simulink model "Fuel_Cell_System"  (R2024a)
settings: Solver=VariableStepAuto  StartTime=0.0  StopTime=10.0  RelTol=1e-3
undefined symbols (not defined in the file): A, Rload
libraries: fl_lib x9, ee_lib x2, nesl_utility x2
settings Model: Creator=Miko  LastModifiedBy=Miko

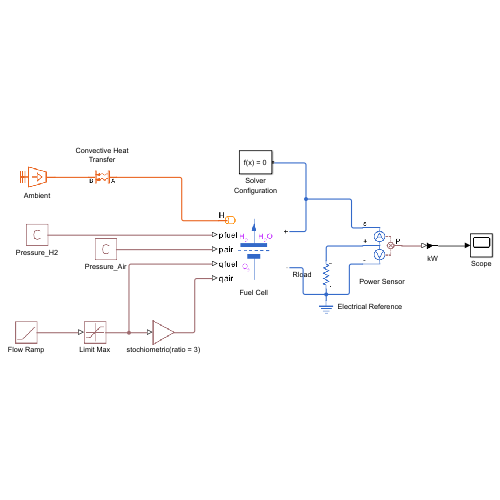
[thumbnail: Simulink's stored preview of the top-level diagram]
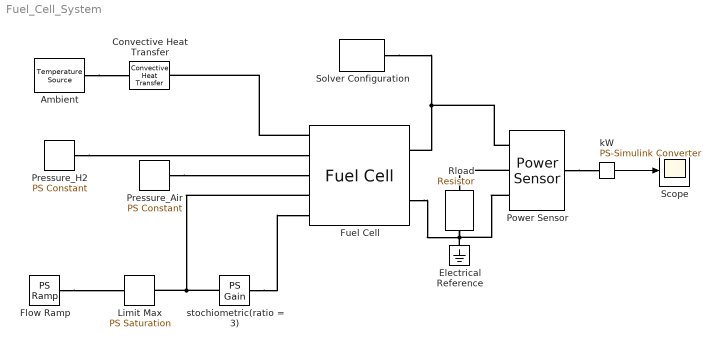
== system Fuel_Cell_System ==
  Ambient : fl_lib/Thermal/Thermal Sources/Temperature Source  temperature=293.15 K
  Convective Heat Transfer : fl_lib/Thermal/Thermal Elements/Convective Heat Transfer  thermal_type=foundation.enum.constant_variable.constant  area=120 cm^2  heat_tr_coeff=20 W/(K*m^2)  min_heat_tr_coeff=1e-3 W/(K*m^2)  T_specify=off  T_priority=None  T=0 K  T_nominal_specify=off  T_nominal_value=1  T_nominal_unit=K  Q_specify=off  Q_priority=None  Q=0 W  Q_nominal_specify=off  Q_nominal_value=1  Q_nominal_unit=W
  Electrical Reference : fl_lib/Electrical/Electrical Elements/Electrical Reference
  Flow Ramp : fl_lib/Physical Signals/Sources/PS Ramp  slope=100/60 lpm/s  start_time=0 s  initial_output=Qfuel0 lpm
  Fuel Cell : ee_lib/Sources/Fuel Cell  model_fidelity=ee.enum.fuelcell.fidelity.detailed  Eoc=Eoc V  A=A V  ri=Ri Ohm  i0=i0 A  i_lim=i_lim A  N_cell=N_cell  number_unit=number_unit  pH2_nom=pH2_nom Pa  pO2_nom=pO2_nom Pa  xH2=99  xO2=21  xW=0  dyn=ee.enum.include.no  Rd=0.005 Ohm  tau=10 s  Tnom=293.15 K  thermal_mass=thermal_mass J/K  iFC_specify=off  iFC_priority=None  iFC=0 A  iFC_nominal_specify=off  iFC_nominal_value=1  iFC_nominal_unit=A  vFC_specify=on  vFC_priority=None  vFC=0 V  vFC_nominal_specify=off  vFC_nominal_value=1  vFC_nominal_unit=V  temperature_specify=on  temperature_priority=High  temperature=293.15 K  temperature_nominal_specify=off  temperature_nominal_value=1  temperature_nominal_unit=K
      settings: InternalSimscapePortConfiguration="{\"Bottom\":[],\"Left\":[{\"id\":\"H\",\"label\":\"H\",\"type\":\"foundation.thermal.thermal\"},{\"id\":\"pfuel\",\"label\":\"pfuel\",\"type\":\"input\"},{\"id\":\"pair\",\"label\":\"pair\",\"type\":\"input\"},{\"id\":\"qfuel\",\"label\":\"qfuel\",\"type\":\"input\"},{\"id\":\"qair\",\"label\":\"qair\",\"type\":\"input\"}],\"Right\":[{\"id\":\"p\",\"label\":\"+\",\"type\":\"foundation.electrical.electrical\"},{\"id\":\"n\",\"label\":\"-\",\"type\":\"foundation.electrical.electrical\"}],\"Top\":[]}"
  Limit Max : fl_lib/Physical Signals/Nonlinear Operators/PS Saturation  upper_limit=100 lpm  lower_limit=0 lpm
  Power Sensor : ee_lib/Sensors & Transducers/Power Sensor  measurement_type=1  averaging_period=1e-4 s
  Pressure_Air : fl_lib/Physical Signals/Sources/PS Constant  constant=1 bar
  Pressure_H2 : fl_lib/Physical Signals/Sources/PS Constant  constant=pH2 bar
  Rload : fl_lib/Electrical/Electrical Elements/Resistor  R=Rload Ohm  i_specify=off  i_priority=None  i=0 A  i_nominal_specify=off  i_nominal_value=1  i_nominal_unit=A  v_specify=off  v_priority=None  v=0 V  v_nominal_specify=off  v_nominal_value=1  v_nominal_unit=V
  Scope : Scope
  Solver Configuration : nesl_utility/Solver Configuration  PhysicalDomain=network_engine_domain  SubClassName=solver  LeftPortType=input  RightPortType=generic  Tones=[]  Harmonics=[]  SimulateNoise=off  Profile=off  UseLocalSampling=off  EnableSwitchedLinearOptims=on  FrequencyDomain=off  UseCCode=off  RelTol=0.001  AbsTol=0.001  MinStep=1e-09  ToWorkspace=off  RevertToSquareIcSolve=off  NumHomotopyIterations=100  PhasorMode=off  PhasorModeNumHarmonics=1  ConsistencySolver=NEWTON_XTOL_AFTER_FTOL  IndexReductionMethod=DerivativeReplacement  DoDC=off  ResidualTolerance=1e-09  ConsistencyTolSource=GLOBAL  ConsistencyAbsTol=0.001  ConsistencyRelTol=0.001  ConsistencyTolFactor=1e-09  UseLocalSolver=off  LocalSolverChoice=NE_BACKWARD_EULER_ADVANCER  ResolveIndetEquations=on  FunctionEvalNumThread=1  LocalSolverSampleTime=0.001  DoFixedCost=off  MaxNonlinIter=3  MaxModeIter=2  ComputeImpulses=off  ImpulseIterations=2  LinearAlgebra=auto  LinearAlgebraNumThread=0  EquationFormulation=NE_TIME_EF  DelaysMemoryBudget=1024  AutomaticFiltering=on  FilteringTimeConstant=0.001  PartitionStorageMethod=AS_NEEDED  PartitionMemoryBudget=1024  PartitionMethod=ROBUST  MultibodyUseLocalSolver=off  MultibodyLocalSolverChoice=ODE1  MultibodyLocalSolverSampleTime=0.001
  kW : nesl_utility/PS-Simulink Converter  PhysicalDomain=network_engine_domain  SubClassName=ps_output  LeftPortType=input  RightPortType=output  PseudoPeriodic=off  Frequencies=[]  VectorFormat=1-D array  Unit=kW  AffineConversion=off
  stochiometric(ratio = 3) : fl_lib/Physical Signals/Functions/PS Gain  gain=3.0
  wires:
  kW/1 -> Scope/1
  connections:
  Fuel Cell/LConn1 -- Convective Heat Transfer/LConn1
  Ambient/LConn1 -- Convective Heat Transfer/RConn1
  Power Sensor/LConn2 -- Rload/LConn1
  Electrical Reference/LConn1 -- Fuel Cell/RConn2 -- Power Sensor/LConn3 -- Rload/RConn1
  Solver Configuration/RConn1 -- Fuel Cell/RConn1 -- Power Sensor/LConn1
  stochiometric(ratio = 3)/LConn1 -- Limit Max/RConn1 -- Fuel Cell/LConn4
  Flow Ramp/RConn1 -- Limit Max/LConn1
  Pressure_Air/RConn1 -- Fuel Cell/LConn3
  Pressure_H2/RConn1 -- Fuel Cell/LConn2
  stochiometric(ratio = 3)/RConn1 -- Fuel Cell/LConn5
  Power Sensor/RConn1 -- kW/LConn1
